simulink model "quadcopter_sim"  (R2023a)
settings: Solver=VariableStepAuto  StartTime=0.0  StopTime=100  RelTol=1e-1
InitFcn:
  | m = 0.0489; % Mass of the drone (kg)
  | d = 0.00116; % Torque constant of one motor (N*m / s^2)
  | b = 4*1e-5; % Thrust constant of one motor (N / s^2)
  | Ixx = 48932*1e-9; % Drone inertia around the xx axis (Kg * m^2)
  | Iyy = 49929*1e-9; % Drone inertia around the yy axis (Kg * m^2)
  | Izz = 99299*1e-9; % Drone inertia around the zz axis (Kg * m^2)
  | l = 0.116 / 2; % Lenght from the motor to the mid point (m)
  | Jr = 729*1e-9; % Rotor inertia (Kg * m^2)
  | Ax = 0; % Air resistance from axis X (kg / s)
  | Ay = 0; % Air resistance from axis Y (kg / s)
  | Az = 0; % Air resistance from axis Z (kg / s)
  | g = 9.81; % The accelaration from gravity (m / s^2)
  | 
  | T_z_acc_low=1/25;
  | Thigh=1/20;
  | Tlow=1/20;
  | 
  | Accel_bias=0;
  | X_dot_dot_bias=0;
  | Y_dot_dot_bias=0;
  | Z_dot_dot_bias=0;
  | Gyro_bias =0;
  | Phi_dot_bias=0;
  | Theta_dot_bias=0;
  | Psi_dot_bias=0;
libraries: slpidlib x4
settings Model: Creator=Artis  LastModifiedBy=tudib
settings OptimizationCC: ReuseModelBlockBuffer=off

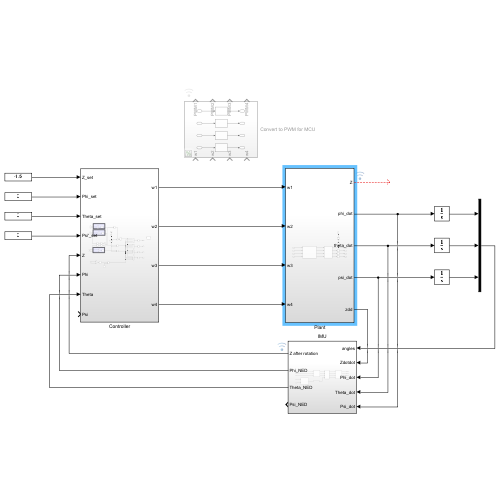
[thumbnail: Simulink's stored preview of the top-level diagram]
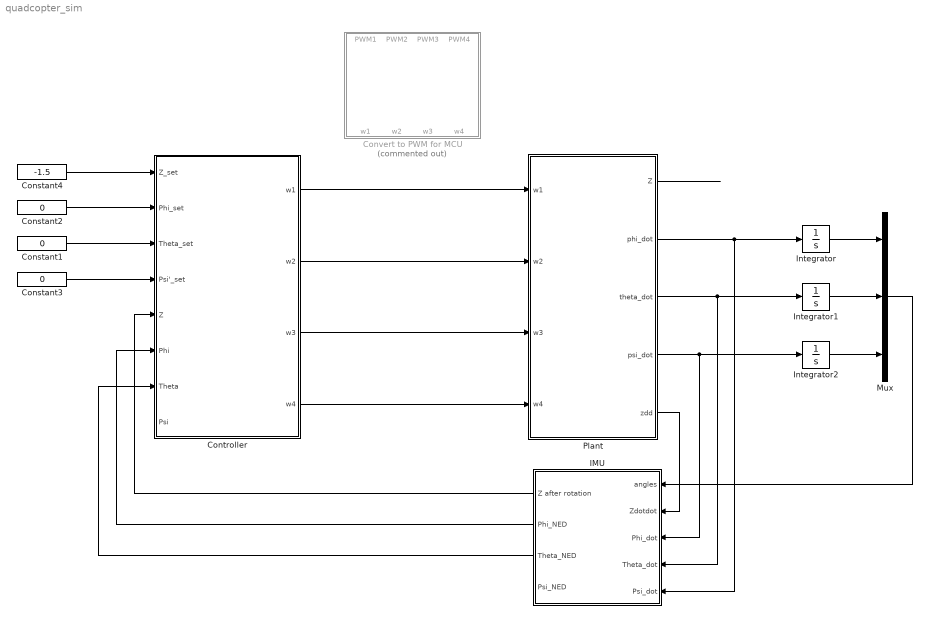
== system quadcopter_sim ==
  Constant1 : Constant  Value=0
  Constant2 : Constant  Value=0
  Constant3 : Constant  Value=0
  Constant4 : Constant  Value=-1.5
  Controller : Subsystem
  Convert to PWM for MCU : Subsystem  Commented=on
  IMU : Subsystem
  Integrator : Integrator
  Integrator1 : Integrator
  Integrator2 : Integrator
  Mux : Mux  Inputs=3
  Plant : Subsystem
  wires:
  Constant2/1 -> Controller/2(Phi_set)
  Constant1/1 -> Controller/3(Theta_set)
  Constant3/1 -> Controller/4(Psi'_set)
  Controller/2(w2) -> Plant/2(w2)
  Controller/4(w4) -> Plant/4(w4)
  Controller/3(w3) -> Plant/3(w3)
  Constant4/1 -> Controller/1(Z_set)
  Controller/1(w1) -> Plant/1(w1)
  IMU/1(Z after rotation) -> Controller/5(Z)
  IMU/2(Phi_NED) -> Controller/6(Phi)
  IMU/3(Theta_NED) -> Controller/7(Theta)
  Plant/4(psi_dot) -> IMU/3(Phi_dot), Integrator2/1
  Plant/3(theta_dot) -> Integrator1/1, IMU/4(Theta_dot)
  Plant/2(phi_dot) -> Integrator/1, IMU/5(Psi_dot)
  Plant/5(zdd) -> IMU/2(Zdotdot)
  Integrator2/1 -> Mux/3
  Integrator1/1 -> Mux/2
  Integrator/1 -> Mux/1
  Mux/1 -> IMU/1(angles)
  Plant/1(Z) -> ?

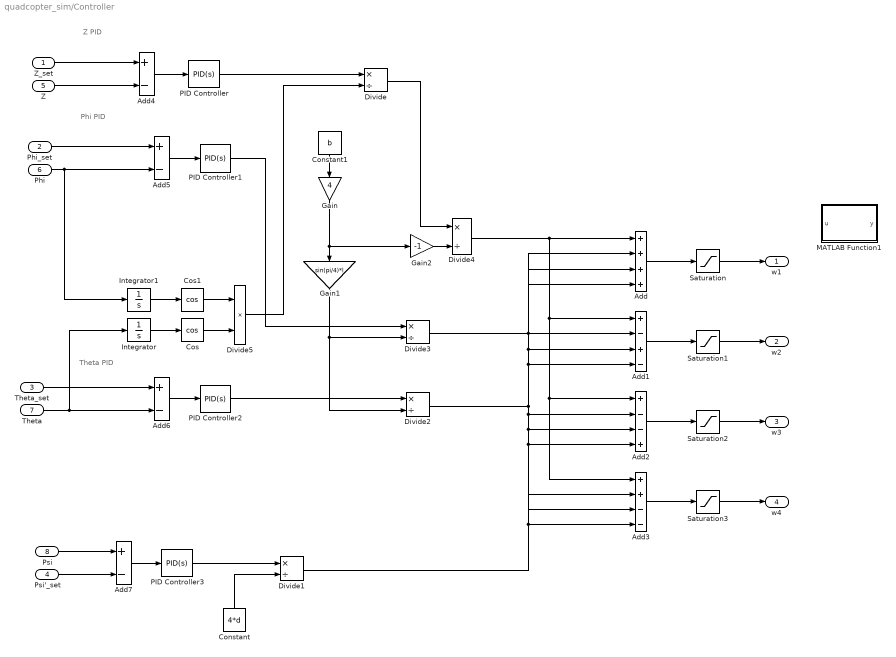
== system quadcopter_sim/Controller ==
  note: Theta PID
  note: Phi PID
  note: Z PID
  Z_set : Inport
  Phi_set : Inport  Port=2
  Theta_set : Inport  Port=3
  Psi'_set : Inport  Port=4
  Z : Inport  Port=5
  Phi : Inport  Port=6
  Theta : Inport  Port=7
  Psi : Inport  Port=8
  Add : Sum  Inputs=++++
  Add1 : Sum  Inputs=+-+-
  Add2 : Sum  Inputs=+--+
  Add3 : Sum  Inputs=++--
  Add{4..7} (4 alike) : Sum  Inputs=+-
  Constant : Constant  Value=4*d
  Constant1 : Constant  Value=b
  Cos : Trigonometry  Operator=cos
  Cos1 : Trigonometry  Operator=cos
  Divide{,1..4} (5 alike) : Product  Inputs=*/
  Divide5 : Product  Inputs=**
  Gain : Gain  Gain=4
  Gain1 : Gain  Gain=sin(pi/4)*l
  Gain2 : Gain  Gain=-1
  Integrator : Integrator
  Integrator1 : Integrator
  MATLAB Function1 : MATLAB Function  TreatAsAtomicUnit=on
  PID Controller : slpidlib/PID Controller  Controller=PID  Form=Parallel  TimeDomain=Continuous-time  UseExternalTs=off  SampleTime=-1  IntegratorMethod=Forward Euler  FilterMethod=Forward Euler  ControllerParametersSource=internal  P=0.6 * 1.7  I=1.2*1.7/3-0.3  UseKiTs=off  D=0.075*1.7*3 - 0.1  N=100  UseFilter=on  TunerSelectOption=Transfer Function Based (PID Tuner App)  InitialConditionSource=internal  InitialConditionForIntegrator=0  InitialConditionForFilter=0  DifferentiatorICPrevScaledInput=0  ExternalReset=none  TrackingMode=off  Kt=1  LimitOutput=off  SatLimitsSource=internal  UpperSaturationLimit=inf  LowerSaturationLimit=-inf  LinearizeAsGain=on  AntiWindupMode=none  Kb=1  LimitIntegrator=off  UpperIntegratorSaturationLimit=inf  LowerIntegratorSaturationLimit=-inf  POutMin=[]  POutMax=[]  IOutMin=[]  IOutMax=[]  DOutMin=[]  DOutMax=[]  NOutMin=[]  NOutMax=[]  SumOutMin=[]  SumOutMax=[]  SaturationOutMin=[]  SaturationOutMax=[]  PParamMin=[]  PParamMax=[]  IParamMin=[]  IParamMax=[]  DParamMin=[]  DParamMax=[]  NParamMin=[]  NParamMax=[]  KbParamMin=[]  KbParamMax=[]  KtParamMin=[]  KtParamMax=[]  KbOutMin=[]  KbOutMax=[]  KtOutMin=[]  KtOutMax=[]  IntegratorOutMin=[]  IntegratorOutMax=[]  FilterOutMin=[]  FilterOutMax=[]  SumI1OutMin=[]  SumI1OutMax=[]  SumI2OutMin=[]  SumI2OutMax=[]  SumI3OutMin=[]  SumI3OutMax=[]  SumI4OutMin=[]  SumI4OutMax=[]  SumDOutMin=[]  SumDOutMax=[]  DifferentiatorOutMin=[]  DifferentiatorOutMax=[]  FilterDiffOutCoefMin=[]  FilterDiffOutCoefMax=[]  ReciprocalOutMin=[]  ReciprocalOutMax=[]  SumDenOutMin=[]  SumDenOutMax=[]  SumNumOutMin=[]  SumNumOutMax=[]  DivideOutMin=[]  DivideOutMax=[]  UdiffTsProdOutMin=[]  UdiffTsProdOutMax=[]  NTsProdOutMin=[]  NTsProdOutMax=[]  UintegralTsProdOutMin=[]  UintegralTsProdOutMax=[]  UngainTsProdOutMin=[]  UngainTsProdOutMax=[]  ClampingZeroOutDataTypeStr=Inherit: Inherit via back propagation  ClampingZeroOutMin=[]  ClampingZeroOutMax=[]  FilterDenConstantOutDataTypeStr=Inherit: Inherit via back propagation  FilterDenConstantOutMin=[]  FilterDenConstantOutMax=[]  PCopyOutDataTypeStr=Inherit: Inherit via back propagation  PCopyOutMin=[]  PCopyOutMax=[]  NCopyOutDataTypeStr=Inherit: Inherit via back propagation  NCopyOutMin=[]  NCopyOutMax=[]  IntegratorContinuousStateAttributes=''  IntegratorStateMustResolveToSignalObject=off  IntegratorRTWStateStorageClass=Auto  FilterContinuousStateAttributes=''  FilterStateMustResolveToSignalObject=off  FilterRTWStateStorageClass=Auto  ParallelPVariant=InternalParameters  IdealPVariant=Disabled  IVariant=InternalParameters  DVariant=InternalParameters  IntegratorVariant=Continuous  SatVariant=Disabled  AWVariant=Passthrough  PCopyVariant=Disabled  TRVariant=Disabled  FdbkBlocksVariant=Forward  IdealPFdbkVariant=Disabled  SatFdbkVariant=Disabled  DerivativeFilterVariant=ContFilter  NVariant=InternalParameters  NCopyVariant=Disabled  FilterICVariant=InternalICsFilter  IntegratorICVariant=InternalICs  ExternalResetVariant=Disabled  TRSumVariant=Passthrough  SumFdbkVariant=Disabled  SumVariant=Sum_PID  TsampFilterVariant=InternalTs  TsampNgainVariant=Passthrough  TsampIntegralVariant=Disabled_SignalSpec  ExternalSaturationOutDataTypeStr=Inherit: Same as second input
  PID Controller1 : slpidlib/PID Controller  Controller=PID  Form=Parallel  TimeDomain=Continuous-time  UseExternalTs=off  SampleTime=-1  IntegratorMethod=Forward Euler  FilterMethod=Forward Euler  ControllerParametersSource=internal  P=-2.29551125806385e-05  I=-1.42052143562565e-06  UseKiTs=off  D=-5.90349375287184e-05  N=1008.51334195282  UseFilter=on  TunerSelectOption=Transfer Function Based (PID Tuner App)  InitialConditionSource=internal  InitialConditionForIntegrator=0  InitialConditionForFilter=0  DifferentiatorICPrevScaledInput=0  ExternalReset=none  TrackingMode=off  Kt=1  LimitOutput=off  SatLimitsSource=internal  UpperSaturationLimit=inf  LowerSaturationLimit=-inf  LinearizeAsGain=on  AntiWindupMode=none  Kb=1  LimitIntegrator=off  UpperIntegratorSaturationLimit=inf  LowerIntegratorSaturationLimit=-inf  POutMin=[]  POutMax=[]  IOutMin=[]  IOutMax=[]  DOutMin=[]  DOutMax=[]  NOutMin=[]  NOutMax=[]  SumOutMin=[]  SumOutMax=[]  SaturationOutMin=[]  SaturationOutMax=[]  PParamMin=[]  PParamMax=[]  IParamMin=[]  IParamMax=[]  DParamMin=[]  DParamMax=[]  NParamMin=[]  NParamMax=[]  KbParamMin=[]  KbParamMax=[]  KtParamMin=[]  KtParamMax=[]  KbOutMin=[]  KbOutMax=[]  KtOutMin=[]  KtOutMax=[]  IntegratorOutMin=[]  IntegratorOutMax=[]  FilterOutMin=[]  FilterOutMax=[]  SumI1OutMin=[]  SumI1OutMax=[]  SumI2OutMin=[]  SumI2OutMax=[]  SumI3OutMin=[]  SumI3OutMax=[]  SumI4OutMin=[]  SumI4OutMax=[]  SumDOutMin=[]  SumDOutMax=[]  DifferentiatorOutMin=[]  DifferentiatorOutMax=[]  FilterDiffOutCoefMin=[]  FilterDiffOutCoefMax=[]  ReciprocalOutMin=[]  ReciprocalOutMax=[]  SumDenOutMin=[]  SumDenOutMax=[]  SumNumOutMin=[]  SumNumOutMax=[]  DivideOutMin=[]  DivideOutMax=[]  UdiffTsProdOutMin=[]  UdiffTsProdOutMax=[]  NTsProdOutMin=[]  NTsProdOutMax=[]  UintegralTsProdOutMin=[]  UintegralTsProdOutMax=[]  UngainTsProdOutMin=[]  UngainTsProdOutMax=[]  ClampingZeroOutDataTypeStr=Inherit: Inherit via back propagation  ClampingZeroOutMin=[]  ClampingZeroOutMax=[]  FilterDenConstantOutDataTypeStr=Inherit: Inherit via back propagation  FilterDenConstantOutMin=[]  FilterDenConstantOutMax=[]  PCopyOutDataTypeStr=Inherit: Inherit via back propagation  PCopyOutMin=[]  PCopyOutMax=[]  NCopyOutDataTypeStr=Inherit: Inherit via back propagation  NCopyOutMin=[]  NCopyOutMax=[]  IntegratorContinuousStateAttributes=''  IntegratorStateMustResolveToSignalObject=off  IntegratorRTWStateStorageClass=Auto  FilterContinuousStateAttributes=''  FilterStateMustResolveToSignalObject=off  FilterRTWStateStorageClass=Auto  ParallelPVariant=InternalParameters  IdealPVariant=Disabled  IVariant=InternalParameters  DVariant=InternalParameters  IntegratorVariant=Continuous  SatVariant=Disabled  AWVariant=Passthrough  PCopyVariant=Disabled  TRVariant=Disabled  FdbkBlocksVariant=Forward  IdealPFdbkVariant=Disabled  SatFdbkVariant=Disabled  DerivativeFilterVariant=ContFilter  NVariant=InternalParameters  NCopyVariant=Disabled  FilterICVariant=InternalICsFilter  IntegratorICVariant=InternalICs  ExternalResetVariant=Disabled  TRSumVariant=Passthrough  SumFdbkVariant=Disabled  SumVariant=Sum_PID  TsampFilterVariant=InternalTs  TsampNgainVariant=Passthrough  TsampIntegralVariant=Disabled_SignalSpec  ExternalSaturationOutDataTypeStr=Inherit: Same as second input
  PID Controller2 : slpidlib/PID Controller  Controller=PID  Form=Parallel  TimeDomain=Continuous-time  UseExternalTs=off  SampleTime=-1  IntegratorMethod=Forward Euler  FilterMethod=Forward Euler  ControllerParametersSource=internal  P=-2.34228279252575e-05  I=-1.44946486469699e-06  UseKiTs=off  D=-6.02377870487898e-05  N=1008.51334195282  UseFilter=on  TunerSelectOption=Transfer Function Based (PID Tuner App)  InitialConditionSource=internal  InitialConditionForIntegrator=0  InitialConditionForFilter=0  DifferentiatorICPrevScaledInput=0  ExternalReset=none  TrackingMode=off  Kt=1  LimitOutput=off  SatLimitsSource=internal  UpperSaturationLimit=inf  LowerSaturationLimit=-inf  LinearizeAsGain=on  AntiWindupMode=none  Kb=1  LimitIntegrator=off  UpperIntegratorSaturationLimit=inf  LowerIntegratorSaturationLimit=-inf  POutMin=[]  POutMax=[]  IOutMin=[]  IOutMax=[]  DOutMin=[]  DOutMax=[]  NOutMin=[]  NOutMax=[]  SumOutMin=[]  SumOutMax=[]  SaturationOutMin=[]  SaturationOutMax=[]  PParamMin=[]  PParamMax=[]  IParamMin=[]  IParamMax=[]  DParamMin=[]  DParamMax=[]  NParamMin=[]  NParamMax=[]  KbParamMin=[]  KbParamMax=[]  KtParamMin=[]  KtParamMax=[]  KbOutMin=[]  KbOutMax=[]  KtOutMin=[]  KtOutMax=[]  IntegratorOutMin=[]  IntegratorOutMax=[]  FilterOutMin=[]  FilterOutMax=[]  SumI1OutMin=[]  SumI1OutMax=[]  SumI2OutMin=[]  SumI2OutMax=[]  SumI3OutMin=[]  SumI3OutMax=[]  SumI4OutMin=[]  SumI4OutMax=[]  SumDOutMin=[]  SumDOutMax=[]  DifferentiatorOutMin=[]  DifferentiatorOutMax=[]  FilterDiffOutCoefMin=[]  FilterDiffOutCoefMax=[]  ReciprocalOutMin=[]  ReciprocalOutMax=[]  SumDenOutMin=[]  SumDenOutMax=[]  SumNumOutMin=[]  SumNumOutMax=[]  DivideOutMin=[]  DivideOutMax=[]  UdiffTsProdOutMin=[]  UdiffTsProdOutMax=[]  NTsProdOutMin=[]  NTsProdOutMax=[]  UintegralTsProdOutMin=[]  UintegralTsProdOutMax=[]  UngainTsProdOutMin=[]  UngainTsProdOutMax=[]  ClampingZeroOutDataTypeStr=Inherit: Inherit via back propagation  ClampingZeroOutMin=[]  ClampingZeroOutMax=[]  FilterDenConstantOutDataTypeStr=Inherit: Inherit via back propagation  FilterDenConstantOutMin=[]  FilterDenConstantOutMax=[]  PCopyOutDataTypeStr=Inherit: Inherit via back propagation  PCopyOutMin=[]  PCopyOutMax=[]  NCopyOutDataTypeStr=Inherit: Inherit via back propagation  NCopyOutMin=[]  NCopyOutMax=[]  IntegratorContinuousStateAttributes=''  IntegratorStateMustResolveToSignalObject=off  IntegratorRTWStateStorageClass=Auto  FilterContinuousStateAttributes=''  FilterStateMustResolveToSignalObject=off  FilterRTWStateStorageClass=Auto  ParallelPVariant=InternalParameters  IdealPVariant=Disabled  IVariant=InternalParameters  DVariant=InternalParameters  IntegratorVariant=Continuous  SatVariant=Disabled  AWVariant=Passthrough  PCopyVariant=Disabled  TRVariant=Disabled  FdbkBlocksVariant=Forward  IdealPFdbkVariant=Disabled  SatFdbkVariant=Disabled  DerivativeFilterVariant=ContFilter  NVariant=InternalParameters  NCopyVariant=Disabled  FilterICVariant=InternalICsFilter  IntegratorICVariant=InternalICs  ExternalResetVariant=Disabled  TRSumVariant=Passthrough  SumFdbkVariant=Disabled  SumVariant=Sum_PID  TsampFilterVariant=InternalTs  TsampNgainVariant=Passthrough  TsampIntegralVariant=Disabled_SignalSpec  ExternalSaturationOutDataTypeStr=Inherit: Same as second input
  PID Controller3 : slpidlib/PID Controller  Controller=PID  Form=Parallel  TimeDomain=Continuous-time  UseExternalTs=off  SampleTime=-1  IntegratorMethod=Forward Euler  FilterMethod=Forward Euler  ControllerParametersSource=internal  P=0  I=0  UseKiTs=off  D=0  N=100  UseFilter=on  TunerSelectOption=Transfer Function Based (PID Tuner App)  InitialConditionSource=internal  InitialConditionForIntegrator=0  InitialConditionForFilter=0  DifferentiatorICPrevScaledInput=0  ExternalReset=none  TrackingMode=off  Kt=1  LimitOutput=off  SatLimitsSource=internal  UpperSaturationLimit=inf  LowerSaturationLimit=-inf  LinearizeAsGain=on  AntiWindupMode=none  Kb=1  LimitIntegrator=off  UpperIntegratorSaturationLimit=inf  LowerIntegratorSaturationLimit=-inf  POutMin=[]  POutMax=[]  IOutMin=[]  IOutMax=[]  DOutMin=[]  DOutMax=[]  NOutMin=[]  NOutMax=[]  SumOutMin=[]  SumOutMax=[]  SaturationOutMin=[]  SaturationOutMax=[]  PParamMin=[]  PParamMax=[]  IParamMin=[]  IParamMax=[]  DParamMin=[]  DParamMax=[]  NParamMin=[]  NParamMax=[]  KbParamMin=[]  KbParamMax=[]  KtParamMin=[]  KtParamMax=[]  KbOutMin=[]  KbOutMax=[]  KtOutMin=[]  KtOutMax=[]  IntegratorOutMin=[]  IntegratorOutMax=[]  FilterOutMin=[]  FilterOutMax=[]  SumI1OutMin=[]  SumI1OutMax=[]  SumI2OutMin=[]  SumI2OutMax=[]  SumI3OutMin=[]  SumI3OutMax=[]  SumI4OutMin=[]  SumI4OutMax=[]  SumDOutMin=[]  SumDOutMax=[]  DifferentiatorOutMin=[]  DifferentiatorOutMax=[]  FilterDiffOutCoefMin=[]  FilterDiffOutCoefMax=[]  ReciprocalOutMin=[]  ReciprocalOutMax=[]  SumDenOutMin=[]  SumDenOutMax=[]  SumNumOutMin=[]  SumNumOutMax=[]  DivideOutMin=[]  DivideOutMax=[]  UdiffTsProdOutMin=[]  UdiffTsProdOutMax=[]  NTsProdOutMin=[]  NTsProdOutMax=[]  UintegralTsProdOutMin=[]  UintegralTsProdOutMax=[]  UngainTsProdOutMin=[]  UngainTsProdOutMax=[]  ClampingZeroOutDataTypeStr=Inherit: Inherit via back propagation  ClampingZeroOutMin=[]  ClampingZeroOutMax=[]  FilterDenConstantOutDataTypeStr=Inherit: Inherit via back propagation  FilterDenConstantOutMin=[]  FilterDenConstantOutMax=[]  PCopyOutDataTypeStr=Inherit: Inherit via back propagation  PCopyOutMin=[]  PCopyOutMax=[]  NCopyOutDataTypeStr=Inherit: Inherit via back propagation  NCopyOutMin=[]  NCopyOutMax=[]  IntegratorContinuousStateAttributes=''  IntegratorStateMustResolveToSignalObject=off  IntegratorRTWStateStorageClass=Auto  FilterContinuousStateAttributes=''  FilterStateMustResolveToSignalObject=off  FilterRTWStateStorageClass=Auto  ParallelPVariant=InternalParameters  IdealPVariant=Disabled  IVariant=InternalParameters  DVariant=InternalParameters  IntegratorVariant=Continuous  SatVariant=Disabled  AWVariant=Passthrough  PCopyVariant=Disabled  TRVariant=Disabled  FdbkBlocksVariant=Forward  IdealPFdbkVariant=Disabled  SatFdbkVariant=Disabled  DerivativeFilterVariant=ContFilter  NVariant=InternalParameters  NCopyVariant=Disabled  FilterICVariant=InternalICsFilter  IntegratorICVariant=InternalICs  ExternalResetVariant=Disabled  TRSumVariant=Passthrough  SumFdbkVariant=Disabled  SumVariant=Sum_PID  TsampFilterVariant=InternalTs  TsampNgainVariant=Passthrough  TsampIntegralVariant=Disabled_SignalSpec  ExternalSaturationOutDataTypeStr=Inherit: Same as second input
  Saturation{,1..3} (4 alike) : Saturate  UpperLimit=3500  LowerLimit=0
  w1 : Outport
  w2 : Outport  Port=2
  w3 : Outport  Port=3
  w4 : Outport  Port=4
  wires:
  Psi/1 -> Add7/1
  Psi'_set/1 -> Add7/2
  Add4/1 -> PID Controller/1
  Integrator/1 -> Cos/1
  Integrator1/1 -> Cos1/1
  Divide5/1 -> Divide/2
  Cos/1 -> Divide5/2
  Constant1/1 -> Gain/1
  Gain/1 -> Gain1/1, Gain2/1
  Gain2/1 -> Divide4/2
  Gain1/1 -> Divide3/2, Divide2/2
  Constant/1 -> Divide1/2
  Divide1/1 -> Add/4, Add1/4, Add2/4, Add3/4
  Divide3/1 -> Add2/2, Add3/2, Add/2, Add1/2
  Divide2/1 -> Add2/3, Add3/3, Add/3, Add1/3
  Divide4/1 -> Add2/1, Add3/1, Add1/1, Add/1
  Add6/1 -> PID Controller2/1
  Add5/1 -> PID Controller1/1
  Divide/1 -> Divide4/1
  Add/1 -> Saturation/1
  Add1/1 -> Saturation1/1
  Add2/1 -> Saturation2/1
  Add3/1 -> Saturation3/1
  Saturation/1 -> w1/1
  Saturation1/1 -> w2/1
  Saturation2/1 -> w3/1
  Saturation3/1 -> w4/1
  Z/1 -> Add4/2
  Z_set/1 -> Add4/1
  Phi/1 -> Add5/2, Integrator1/1
  Phi_set/1 -> Add5/1
  Theta/1 -> Add6/2, Integrator/1
  Theta_set/1 -> Add6/1
  PID Controller/1 -> Divide/1
  PID Controller1/1 -> Divide3/1
  PID Controller2/1 -> Divide2/1
  Cos1/1 -> Divide5/1
  Add7/1 -> PID Controller3/1
  PID Controller3/1 -> Divide1/1

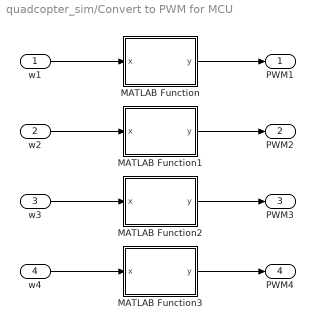
== system quadcopter_sim/Convert to PWM for MCU ==
  w1 : Inport
  w2 : Inport  Port=2
  w3 : Inport  Port=3
  w4 : Inport  Port=4
  MATLAB Function : MATLAB Function  TreatAsAtomicUnit=on
  MATLAB Function1 : MATLAB Function  TreatAsAtomicUnit=on
  MATLAB Function2 : MATLAB Function  TreatAsAtomicUnit=on
  MATLAB Function3 : MATLAB Function  TreatAsAtomicUnit=on
  PWM1 : Outport
  PWM2 : Outport  Port=2
  PWM3 : Outport  Port=3
  PWM4 : Outport  Port=4
  wires:
  MATLAB Function1/1(y) -> PWM2/1
  w1/1 -> MATLAB Function/1(x)
  w3/1 -> MATLAB Function2/1(x)
  w2/1 -> MATLAB Function1/1(x)
  MATLAB Function2/1(y) -> PWM3/1
  MATLAB Function/1(y) -> PWM1/1
  MATLAB Function3/1(y) -> PWM4/1
  w4/1 -> MATLAB Function3/1(x)

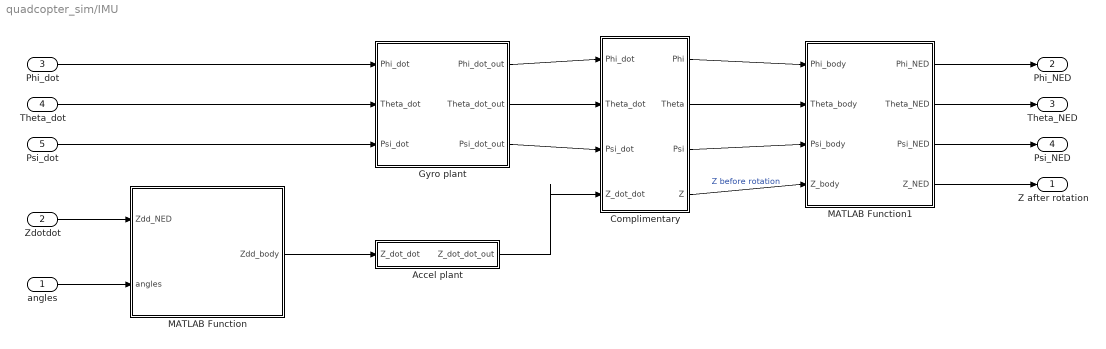
== system quadcopter_sim/IMU ==
  angles : Inport
  Zdotdot : Inport  Port=2
  Phi_dot : Inport  Port=3
  Theta_dot : Inport  Port=4
  Psi_dot : Inport  Port=5
  Accel plant : Subsystem
  Complimentary : Subsystem
  Gyro plant : Subsystem
  MATLAB Function : MATLAB Function  TreatAsAtomicUnit=on
  MATLAB Function1 : MATLAB Function  TreatAsAtomicUnit=on
  Z after rotation : Outport
  Phi_NED : Outport  Port=2
  Theta_NED : Outport  Port=3
  Psi_NED : Outport  Port=4
  wires:
  Accel plant/1(Z_dot_dot_out) -> Complimentary/4(Z_dot_dot)
  MATLAB Function/1(Zdd_body) -> Accel plant/1(Z_dot_dot)
  Gyro plant/1(Phi_dot_out) -> Complimentary/1(Phi_dot)
  Gyro plant/2(Theta_dot_out) -> Complimentary/2(Theta_dot)
  angles/1 -> MATLAB Function/2(angles)
  Complimentary/1(Phi) -> MATLAB Function1/1(Phi_body)
  Gyro plant/3(Psi_dot_out) -> Complimentary/3(Psi_dot)
  Complimentary/3(Psi) -> MATLAB Function1/3(Psi_body)
  Complimentary/4(Z) -> MATLAB Function1/4(Z_body)  "Z before rotation"
  Complimentary/2(Theta) -> MATLAB Function1/2(Theta_body)
  Psi_dot/1 -> Gyro plant/3(Psi_dot)
  Theta_dot/1 -> Gyro plant/2(Theta_dot)
  MATLAB Function1/1(Phi_NED) -> Phi_NED/1
  MATLAB Function1/2(Theta_NED) -> Theta_NED/1
  Phi_dot/1 -> Gyro plant/1(Phi_dot)
  Zdotdot/1 -> MATLAB Function/1(Zdd_NED)
  MATLAB Function1/3(Psi_NED) -> Psi_NED/1
  MATLAB Function1/4(Z_NED) -> Z after rotation/1

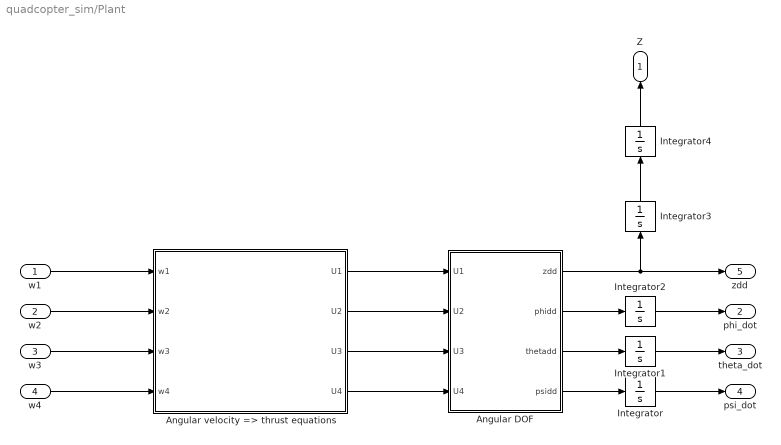
== system quadcopter_sim/Plant ==
  w1 : Inport
  w2 : Inport  Port=2
  w3 : Inport  Port=3
  w4 : Inport  Port=4
  Angular DOF : Subsystem
  Angular velocity => thrust equations : Subsystem
  Integrator{,1..3} (4 alike) : Integrator
  Integrator4 : Integrator  LimitOutput=on  UpperSaturationLimit=0
  Z : Outport
  phi_dot : Outport  Port=2
  theta_dot : Outport  Port=3
  psi_dot : Outport  Port=4
  zdd : Outport  Port=5
  wires:
  w1/1 -> Angular velocity => thrust equations/1(w1)
  w3/1 -> Angular velocity => thrust equations/3(w3)
  Angular velocity => thrust equations/4(U4) -> Angular DOF/4(U4)
  Angular velocity => thrust equations/3(U3) -> Angular DOF/3(U3)
  Angular velocity => thrust equations/2(U2) -> Angular DOF/2(U2)
  w2/1 -> Angular velocity => thrust equations/2(w2)
  w4/1 -> Angular velocity => thrust equations/4(w4)
  Angular velocity => thrust equations/1(U1) -> Angular DOF/1(U1)
  Angular DOF/4(psidd) -> Integrator/1
  Angular DOF/3(thetadd) -> Integrator1/1
  Angular DOF/2(phidd) -> Integrator2/1
  Angular DOF/1(zdd) -> Integrator3/1, zdd/1
  Integrator2/1 -> phi_dot/1
  Integrator1/1 -> theta_dot/1
  Integrator/1 -> psi_dot/1
  Integrator3/1 -> Integrator4/1
  Integrator4/1 -> Z/1

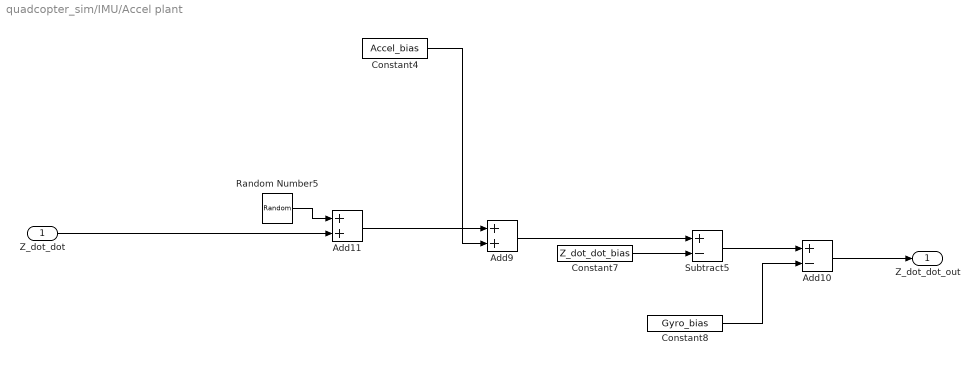
== system quadcopter_sim/IMU/Accel plant ==
  Z_dot_dot : Inport
  Add10 : Sum  Inputs=+-
  Add11 : Sum
  Add9 : Sum
  Constant4 : Constant  Value=Accel_bias
  Constant7 : Constant  Value=Z_dot_dot_bias
  Constant8 : Constant  Value=Gyro_bias
  Random Number5 : RandomNumber  Variance=0.0001  Seed=1  SampleTime=0.001
  Subtract5 : Sum  Inputs=+-
  Z_dot_dot_out : Outport
  wires:
  Subtract5/1 -> Add10/1
  Add9/1 -> Subtract5/1
  Constant4/1 -> Add9/2
  Random Number5/1 -> Add11/1
  Z_dot_dot/1 -> Add11/2
  Constant7/1 -> Subtract5/2
  Add11/1 -> Add9/1
  Constant8/1 -> Add10/2
  Add10/1 -> Z_dot_dot_out/1

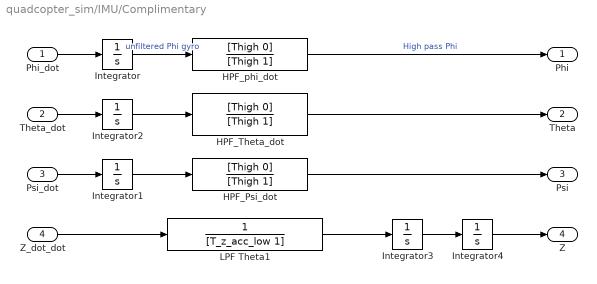
== system quadcopter_sim/IMU/Complimentary ==
  Phi_dot : Inport
  Theta_dot : Inport  Port=2
  Psi_dot : Inport  Port=3
  Z_dot_dot : Inport  Port=4
  HPF_Psi_dot : TransferFcn  Numerator=[Thigh 0]  Denominator=[Thigh 1]
  HPF_Theta_dot : TransferFcn  Numerator=[Thigh 0]  Denominator=[Thigh 1]
  HPF_phi_dot : TransferFcn  Numerator=[Thigh 0]  Denominator=[Thigh 1]
  Integrator{,1..3} (4 alike) : Integrator
  Integrator4 : Integrator  LimitOutput=on  UpperSaturationLimit=0
  LPF Theta1 : TransferFcn  Denominator=[T_z_acc_low 1]
  Phi : Outport
  Theta : Outport  Port=2
  Psi : Outport  Port=3
  Z : Outport  Port=4
  wires:
  Phi_dot/1 -> Integrator/1
  Theta_dot/1 -> Integrator2/1
  Psi_dot/1 -> Integrator1/1
  Z_dot_dot/1 -> LPF Theta1/1
  Integrator/1 -> HPF_phi_dot/1  "unfiltered Phi gyro"
  Integrator2/1 -> HPF_Theta_dot/1
  Integrator1/1 -> HPF_Psi_dot/1
  HPF_Theta_dot/1 -> Theta/1
  HPF_Psi_dot/1 -> Psi/1
  HPF_phi_dot/1 -> Phi/1  "High pass Phi"
  Integrator4/1 -> Z/1
  Integrator3/1 -> Integrator4/1
  LPF Theta1/1 -> Integrator3/1

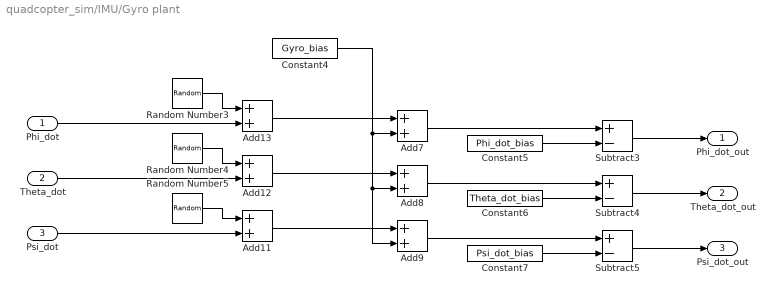
== system quadcopter_sim/IMU/Gyro plant ==
  Phi_dot : Inport
  Theta_dot : Inport  Port=2
  Psi_dot : Inport  Port=3
  Add{7..9,11..13} (6 alike) : Sum
  Constant4 : Constant  Value=Gyro_bias
  Constant5 : Constant  Value=Phi_dot_bias
  Constant6 : Constant  Value=Theta_dot_bias
  Constant7 : Constant  Value=Psi_dot_bias
  Random Number3 : RandomNumber  Variance=0.0001  Seed=1  SampleTime=0.001
  Random Number4 : RandomNumber  Variance=0.0001  Seed=1  SampleTime=0.001
  Random Number5 : RandomNumber  Variance=0.0001  Seed=1  SampleTime=0.001
  Subtract3 : Sum  Inputs=+-
  Subtract4 : Sum  Inputs=+-
  Subtract5 : Sum  Inputs=+-
  Phi_dot_out : Outport
  Theta_dot_out : Outport  Port=2
  Psi_dot_out : Outport  Port=3
  wires:
  Subtract4/1 -> Theta_dot_out/1
  Add7/1 -> Subtract3/1
  Add12/1 -> Add8/1
  Add9/1 -> Subtract5/1
  Add8/1 -> Subtract4/1
  Constant4/1 -> Add7/2, Add9/2, Add8/2
  Constant5/1 -> Subtract3/2
  Subtract3/1 -> Phi_dot_out/1
  Constant6/1 -> Subtract4/2
  Random Number5/1 -> Add11/1
  Psi_dot/1 -> Add11/2
  Phi_dot/1 -> Add13/2
  Random Number4/1 -> Add12/1
  Constant7/1 -> Subtract5/2
  Theta_dot/1 -> Add12/2
  Random Number3/1 -> Add13/1
  Add13/1 -> Add7/1
  Add11/1 -> Add9/1
  Subtract5/1 -> Psi_dot_out/1

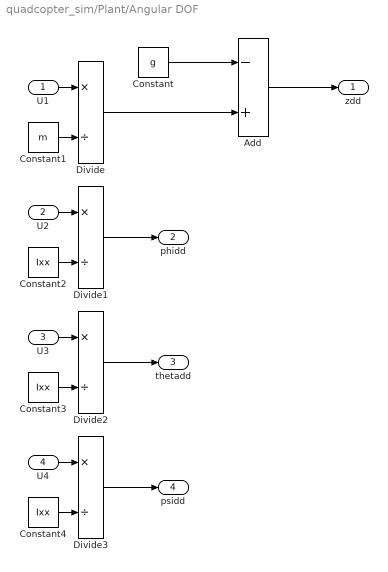
== system quadcopter_sim/Plant/Angular DOF ==
  U1 : Inport
  U2 : Inport  Port=2
  U3 : Inport  Port=3
  U4 : Inport  Port=4
  Add : Sum  Inputs=-+
  Constant : Constant  Value=g
  Constant1 : Constant  Value=m
  Constant2 : Constant  Value=Ixx
  Constant3 : Constant  Value=Ixx
  Constant4 : Constant  Value=Ixx
  Divide{,1..3} (4 alike) : Product  Inputs=*/
  zdd : Outport
  phidd : Outport  Port=2
  thetadd : Outport  Port=3
  psidd : Outport  Port=4
  wires:
  Constant/1 -> Add/1
  U1/1 -> Divide/1
  Constant1/1 -> Divide/2
  Divide/1 -> Add/2
  Add/1 -> zdd/1
  U2/1 -> Divide1/1
  Constant2/1 -> Divide1/2
  Constant3/1 -> Divide2/2
  U3/1 -> Divide2/1
  U4/1 -> Divide3/1
  Constant4/1 -> Divide3/2
  Divide1/1 -> phidd/1
  Divide2/1 -> thetadd/1
  Divide3/1 -> psidd/1

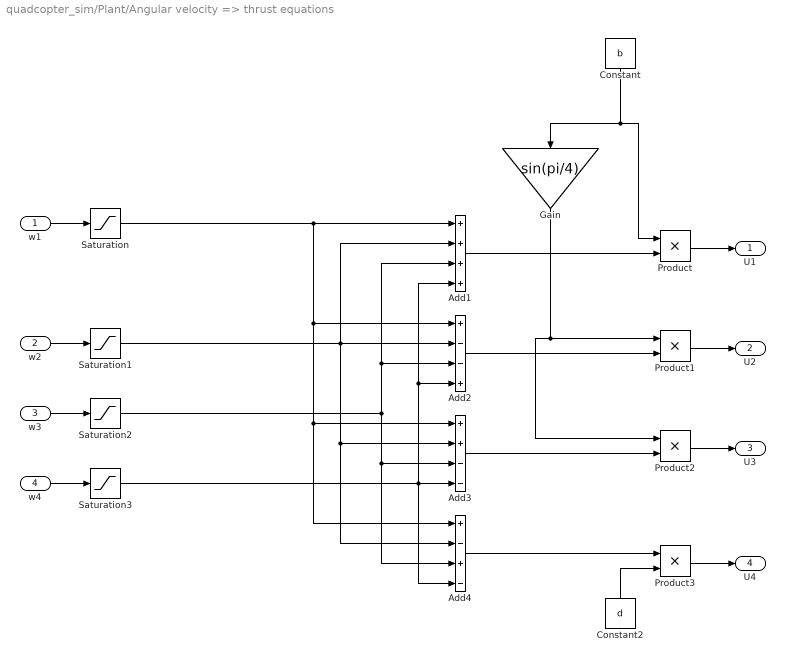
== system quadcopter_sim/Plant/Angular velocity => thrust equations ==
  w1 : Inport
  w2 : Inport  Port=2
  w3 : Inport  Port=3
  w4 : Inport  Port=4
  Add1 : Sum  Inputs=++++
  Add2 : Sum  Inputs=+--+
  Add3 : Sum  Inputs=++--
  Add4 : Sum  Inputs=+-+-
  Constant : Constant  Value=b
  Constant2 : Constant  Value=d
  Gain : Gain  Gain=sin(pi/4)
  Product{,1..3} (4 alike) : Product
  Saturation{,1..3} (4 alike) : Saturate  UpperLimit=inf  LowerLimit=0
  U1 : Outport
  U2 : Outport  Port=2
  U3 : Outport  Port=3
  U4 : Outport  Port=4
  wires:
  w1/1 -> Saturation/1
  w2/1 -> Saturation1/1
  w3/1 -> Saturation2/1
  w4/1 -> Saturation3/1
  Product/1 -> U1/1
  Add1/1 -> Product/2
  Add4/1 -> Product3/1
  Add3/1 -> Product2/2
  Add2/1 -> Product1/2
  Constant2/1 -> Product3/2
  Gain/1 -> Product2/1, Product1/1
  Product3/1 -> U4/1
  Product2/1 -> U3/1
  Product1/1 -> U2/1
  Constant/1 -> Product/1, Gain/1
  Saturation/1 -> Add1/1, Add2/1, Add3/1, Add4/1
  Saturation1/1 -> Add3/2, Add4/2, Add2/2, Add1/2
  Saturation2/1 -> Add1/3, Add2/3, Add3/3, Add4/3
  Saturation3/1 -> Add4/4, Add2/4, Add1/4, Add3/4

== matlab function quadcopter_sim/Convert to PWM for MCU/MATLAB Function1 ==
  data: x input; y output
function y = fcn(x)

y =  8.679e-15*x^9 -9.4e-12*x^8 + 4.063e-09*x^7 -8.819e-07*x^6 + 9.718e-05*x^5 -0.004292*x^4 -0.07222*x^3 + 10.47*x^2 + 30.47*x -1161;

== matlab function quadcopter_sim/Convert to PWM for MCU/MATLAB Function2 ==
  data: x input; y output
function y = fcn(x)

y =  8.679e-15*x^9 -9.4e-12*x^8 + 4.063e-09*x^7 -8.819e-07*x^6 + 9.718e-05*x^5 -0.004292*x^4 -0.07222*x^3 + 10.47*x^2 + 30.47*x -1161;

== matlab function quadcopter_sim/Convert to PWM for MCU/MATLAB Function3 ==
  data: x input; y output
function y = fcn(x)

y =  8.679e-15*x^9 -9.4e-12*x^8 + 4.063e-09*x^7 -8.819e-07*x^6 + 9.718e-05*x^5 -0.004292*x^4 -0.07222*x^3 + 10.47*x^2 + 30.47*x -1161;

== matlab function quadcopter_sim/IMU/MATLAB Function1 ==
  data: Phi_NED output; Theta_NED output; Psi_NED output; Phi_body input; Theta_body input; Psi_body input; Z_body input; Z_NED output
function [Phi_NED, Theta_NED, Psi_NED, Z_NED] = BODYtoNED(Phi_body, Theta_body, Psi_body, Z_body)

F=-Phi_body;
T=-Theta_body;
P=-Psi_body;



Phi_NED = Psi_body*(sin(F)*sin(P) - cos(F)*cos(P)*sin(T)) + Theta_body*(cos(F)*sin(P) + cos(P)*sin(F)*sin(T)) + Phi_body*cos(P)*cos(T);
Theta_NED = Psi_body*(cos(P)*sin(F) + cos(F)*sin(P)*sin(T)) + Theta_body*(cos(F)*cos(P) - sin(F)*sin(P)*sin(T)) - Phi_body*cos(T)*sin(P);
Psi_NED = Phi_body*sin(T) + Psi_body*cos(F)*cos(T) - Theta_body*cos(T)*sin(F);


Z_NED = Z_body*cos(F)*cos(T);

== matlab function quadcopter_sim/IMU/MATLAB Function ==
  data: Zdd_body output; Zdd_NED input; angles input
function Zdd_body  = NEDtoBODY(Zdd_NED, angles)

Phi=angles(1);
Theta=angles(2);
Psi=angles(3);

Zdd_body=Zdd_NED*cos(Phi)*cos(Theta);

== matlab function quadcopter_sim/Controller/MATLAB Function1 ==
  data: u input; y output
function y = fcn(u)
    if 0.0795*u - 21.961 > 255
        q = 255;
    elseif 0.0795*u - 21.961 < 0
        q = 0;
    else
        q = (0.0795*u - 21.961);
    end
y = q;

== matlab function quadcopter_sim/Convert to PWM for MCU/MATLAB Function ==
  data: x input; y output
function y = fcn(x)

y =  8.679e-15*x^9 -9.4e-12*x^8 + 4.063e-09*x^7 -8.819e-07*x^6 + 9.718e-05*x^5 -0.004292*x^4 -0.07222*x^3 + 10.47*x^2 + 30.47*x -1161;
